simulink library "amg_high_precision_rtc"  (R2015b)
settings: Solver=ode45  StartTime=0.0  StopTime=10.0  RelTol=1e-3
libraries: simulink x207, waijung_soft_i2c_lib x11, amg_high_precision_rtc x10
(part 3 of 5)

== system amg_high_precision_rtc/STM32F4/DS3231 Get Time/Convert/Convert Hour ==
  In1 : Inport
  Add : Sum
  Constant : Constant  Value=10  OutDataTypeStr=uint8
  Extract Bits : simulink/Logic and Bit Operations/Extract Bits  SystemSampleTime=-1  bitsToExtract=Range of bits  numBits=8  bitIdxRange=[4 5]  outScalingMode=Treat bit field as an integer
  Extract Bits1 : simulink/Logic and Bit Operations/Extract Bits  SystemSampleTime=-1  bitsToExtract=Range of bits  numBits=8  bitIdxRange=[0 3]  outScalingMode=Treat bit field as an integer
  Extract Bits2 : simulink/Logic and Bit Operations/Extract Bits  SystemSampleTime=-1  bitsToExtract=Range of bits  numBits=8  bitIdxRange=[5 5]  outScalingMode=Treat bit field as an integer
  Product : Product  RndMeth=Zero
  Hour : Outport
  AM/PM : Outport  Port=2
  wires:
  Add/1 -> Hour/1
  Product/1 -> Add/1
  Extract Bits/1 -> Product/2
  Constant/1 -> Product/1
  In1/1 -> Extract Bits/1, Extract Bits1/1, Extract Bits2/1
  Extract Bits1/1 -> Add/2
  Extract Bits2/1 -> AM/PM/1

== system amg_high_precision_rtc/STM32F4/DS3231 Get Time/Convert/Convert Second// Minute ==
  In1 : Inport
  Add : Sum
  Constant : Constant  Value=10  OutDataTypeStr=uint8
  Extract Bits : simulink/Logic and Bit Operations/Extract Bits  SystemSampleTime=-1  bitsToExtract=Range of bits  numBits=8  bitIdxRange=[4 6]  outScalingMode=Treat bit field as an integer
  Extract Bits1 : simulink/Logic and Bit Operations/Extract Bits  SystemSampleTime=-1  bitsToExtract=Range of bits  numBits=8  bitIdxRange=[0 3]  outScalingMode=Treat bit field as an integer
  Product : Product  RndMeth=Zero
  Out1 : Outport
  wires:
  In1/1 -> Extract Bits/1, Extract Bits1/1
  Constant/1 -> Product/1
  Extract Bits/1 -> Product/2
  Product/1 -> Add/1
  Extract Bits1/1 -> Add/2
  Add/1 -> Out1/1

== system amg_high_precision_rtc/STM32F4/DS3231Temperture/Check Busy// Write Conv/If Action Active CONV ==
  In1 : Inport
  Action Port : ActionPort  PropagateVarSize=During execution  ActionType=then
  CONV : Constant  Value=hex2dec('3C')  OutDataTypeStr=uint8
  I2C Master Read/Write1 : S-Function  FunctionName=stm32f4_i2c  Parameters=configuration,module,transfer,clkspeed,timeout,sdapin,sclpin,writecount,readcount,inputtypearray,outputtypearray,confstr,sampletime,sampletimestr,blockid  SFunctionDeploymentMode=off  EnableBusSupport=off  mask(stm32f4_i2c){configuration=Transaction, module=1, lastmodule=3, transfer=Blocking, dutycycle=TLow/THigh = 2, clkspeed=400, timeout=25, writecount=2, readcount=0, sdapin=C9, sclpin=A8, waitwritetime=0, inputtypearray=[3 3 3 3], outputtypearray=[1 3], confstr=["C","9","A","8","1","1","6","0","I2C_DutyCycle_2","0"], sampletime=-1, sampletimestr=0, blockid=amg_high_precision_rtcTempertureReadSubsystemIfActionSubsystemI2CMasterReadWrite1}
      mask prompts: module "I2C Module"; lastmodule "Last module"; transfer "Transfer mode"; dutycycle "Duty cycle in fast mode"; clkspeed "Clock speed (kHz)"; timeout "Timeout (ms)"; writecount "Bytes write count"; readcount "Bytes read count"; sdapin "SDA pin"; sclpin "SCL pin"; waitwritetime "Wait write time (ms), default is 0"; inputtypearray "Input type array"; outputtypearray "Output type array"; confstr "Configuration string"; sampletime "Sample time (sec)"; sampletimestr "Compiled sample time (sec) in string"
      mask init:
      | stm32f4_i2c_callback('init');
      mask Help: web(fullfile(waijungdocroot,'stm32f4_i2c_readwrite.htm'), '-browser')
      mask TypeOptions configuration: Setup | Transaction
      mask Callback configuration: stm32f4_i2c_callback('configuration');
      mask TypeOptions module: 1 | 2 | 3
      mask Callback module: stm32f4_i2c_callback('module');
      mask TypeOptions transfer: Blocking | Non-blocking
      mask TypeOptions dutycycle: TLow/THigh = 16/9 | TLow/THigh = 2
      mask Callback dutycycle: stm32f4_i2c_callback('dutycycle');
      mask Callback writecount: stm32f4_i2c_callback('writecount');
      mask Callback readcount: stm32f4_i2c_callback('readcount');
      mask TypeOptions sdapin: - | C9
      mask Callback sdapin: stm32f4_i2c_callback('sdapin');
      mask TypeOptions sclpin: - | A8
      mask Callback sclpin: stm32f4_i2c_callback('sclpin');
      mask Callback confstr: stm32f4_i2c_callback('confstr');
      mask Callback sampletime: stm32f4_i2c_callback('sampletime');
      mask Callback sampletimestr: stm32f4_i2c_callback('sampletimestr');
      mask Callback blockid: stm32f4_i2c_callback('blockid');
      mask Display: text(0.5, 0.5, 'Module: I2C1\nTransfer: Blocking\nWrite: 2 bytes\nRead: 0 bytes\nTs (sec): 0','ver','middle','hor','center');port_label('input', 1,'SlvAddr');port_label('input', 2,'Wr0 (uint8)');port_label('input', 3,'Wr1 (uint8)');port_label('output', 1,'Status');
  REG_CNTRL : Constant  Value=hex2dec('0E')  OutDataTypeStr=uint8
  Terminator : Terminator
  wires:
  In1/1 -> I2C Master Read/Write1/1
  CONV/1 -> I2C Master Read/Write1/3
  REG_CNTRL/1 -> I2C Master Read/Write1/2
  I2C Master Read/Write1/1 -> Terminator/1

== system amg_high_precision_rtc/Soft I2C/Soft-DS3231 Configure/Debouce4/Enabled Subsystem ==
  Enable : EnablePort  PropagateVarSize=During execution
  Counter Free-Running : simulink/Sources/Counter Free-Running  SystemSampleTime=-1  NumBits=32  tsamp=-1
  Out1 : Outport  InitialOutput=0
  wires:
  Counter Free-Running/1 -> Out1/1

== system amg_high_precision_rtc/Soft I2C/Soft-DS3231 Configure/Debouce4/Enabled Subsystem1 ==
  Enable : EnablePort  PropagateVarSize=During execution
  Bitwise Operator : simulink/Logic and Bit Operations/Bitwise Operator  logicop=AND  UseBitMask=on  BitMask=1  BitMaskRealWorld=Stored Integer
  Compare To Zero : simulink/Logic and Bit Operations/Compare To Zero  SystemSampleTime=-1  relop===  LogicOutDataTypeMode=uint8  ZeroCross=off
  Counter Free-Running : simulink/Sources/Counter Free-Running  SystemSampleTime=-1  NumBits=32  tsamp=-1
  Out1 : Outport  InitialOutput=0
  wires:
  Compare To Zero/1 -> Out1/1
  Bitwise Operator/1 -> Compare To Zero/1
  Counter Free-Running/1 -> Bitwise Operator/1

== system amg_high_precision_rtc/Soft I2C/Soft-DS3231 Configure/Debouce4/Enabled Subsystem4 ==
  Enable : EnablePort  PropagateVarSize=During execution
  Counter Free-Running : simulink/Sources/Counter Free-Running  SystemSampleTime=-1  NumBits=32  tsamp=-1
  Out1 : Outport  InitialOutput=0
  wires:
  Counter Free-Running/1 -> Out1/1

== system amg_high_precision_rtc/Soft I2C/Soft-DS3231 Configure/Debouce4/Enabled Subsystem5 ==
  Enable : EnablePort  PropagateVarSize=During execution
  Counter Free-Running : simulink/Sources/Counter Free-Running  SystemSampleTime=-1  NumBits=32  tsamp=-1
  Out1 : Outport  InitialOutput=0
  wires:
  Counter Free-Running/1 -> Out1/1

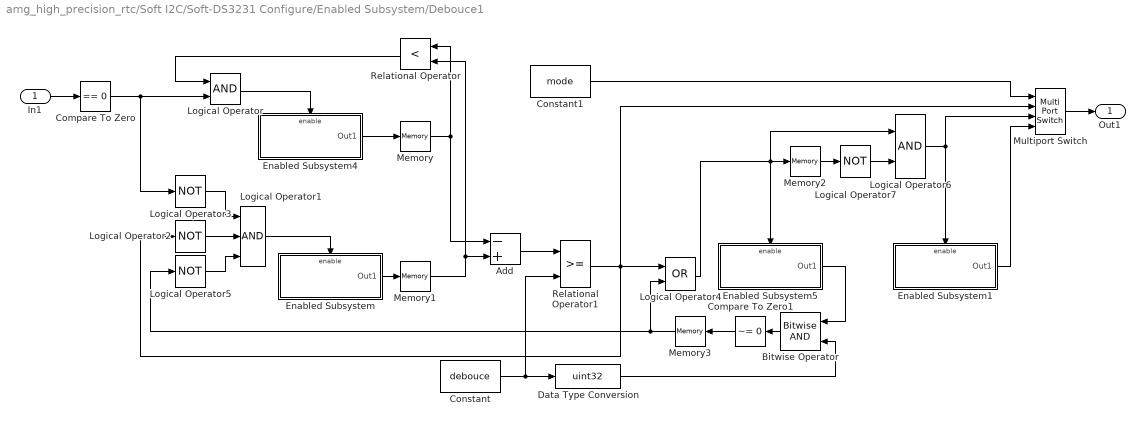
== system amg_high_precision_rtc/Soft I2C/Soft-DS3231 Configure/Enabled Subsystem/Debouce1 ==
  In1 : Inport
  Add : Sum  Inputs=-+  OutDataTypeStr=int32
  Bitwise Operator : simulink/Logic and Bit Operations/Bitwise Operator  logicop=AND  UseBitMask=off  NumInputPorts=2  BitMask=debouce  BitMaskRealWorld=Stored Integer
  Compare To Zero : simulink/Logic and Bit Operations/Compare To Zero  SystemSampleTime=-1  relop===  LogicOutDataTypeMode=uint8  ZeroCross=off
  Compare To Zero1 : simulink/Logic and Bit Operations/Compare To Zero  SystemSampleTime=-1  relop=~=  LogicOutDataTypeMode=boolean  ZeroCross=off
  Constant : Constant  Value=debouce  OutDataTypeStr=int32
  Constant1 : Constant  Value=mode  OutDataTypeStr=int32
  Data Type Conversion : DataTypeConversion  OutDataTypeStr=uint32
  Enabled Subsystem : Subsystem  TreatAsAtomicUnit=on
  Enabled Subsystem1 : Subsystem  TreatAsAtomicUnit=on
  Enabled Subsystem4 : Subsystem  TreatAsAtomicUnit=on
  Enabled Subsystem5 : Subsystem  TreatAsAtomicUnit=on
  Logical Operator : Logic  AllPortsSameDT=off  OutDataTypeStr=boolean
  Logical Operator1 : Logic  Inputs=3  AllPortsSameDT=off  OutDataTypeStr=boolean
  Logical Operator{2..3,5,7} (4 alike) : Logic  Operator=NOT  AllPortsSameDT=off  OutDataTypeStr=boolean
  Logical Operator4 : Logic  Operator=OR  AllPortsSameDT=off  OutDataTypeStr=boolean
  Logical Operator6 : Logic  AllPortsSameDT=off  OutDataTypeStr=boolean
  Memory{,1..3} (4 alike) : Memory  LinearizeMemory=on
  Multiport Switch : MultiPortSwitch
  Relational Operator : RelationalOperator  Operator=<  OutDataTypeStr=boolean
  Relational Operator1 : RelationalOperator  OutDataTypeStr=boolean  InputSameDT=on
  Out1 : Outport
  wires:
  Logical Operator1/1 -> Enabled Subsystem/Enable
  Relational Operator1/1 -> Logical Operator2/1, Logical Operator4/1, Multiport Switch/2
  Logical Operator7/1 -> Logical Operator6/2
  Memory2/1 -> Logical Operator7/1
  Logical Operator4/1 -> Logical Operator6/1, Memory2/1, Enabled Subsystem5/Enable
  Enabled Subsystem5/1(Out1) -> Bitwise Operator/1
  Bitwise Operator/1 -> Compare To Zero1/1
  Compare To Zero1/1 -> Memory3/1
  Logical Operator3/1 -> Logical Operator1/1
  Logical Operator5/1 -> Logical Operator1/3
  Memory3/1 -> Logical Operator5/1, Logical Operator4/2
  Logical Operator2/1 -> Logical Operator1/2
  Constant/1 -> Relational Operator1/2, Data Type Conversion/1
  Add/1 -> Relational Operator1/1
  Relational Operator/1 -> Logical Operator/1
  Logical Operator/1 -> Enabled Subsystem4/Enable
  Compare To Zero/1 -> Logical Operator3/1, Logical Operator/2
  Memory1/1 -> Relational Operator/2, Add/2
  Memory/1 -> Add/1, Relational Operator/1
  Enabled Subsystem4/1(Out1) -> Memory/1
  Enabled Subsystem/1(Out1) -> Memory1/1
  In1/1 -> Compare To Zero/1
  Logical Operator6/1 -> Multiport Switch/3, Enabled Subsystem1/Enable
  Enabled Subsystem1/1(Out1) -> Multiport Switch/4
  Data Type Conversion/1 -> Bitwise Operator/2
  Multiport Switch/1 -> Out1/1
  Constant1/1 -> Multiport Switch/1

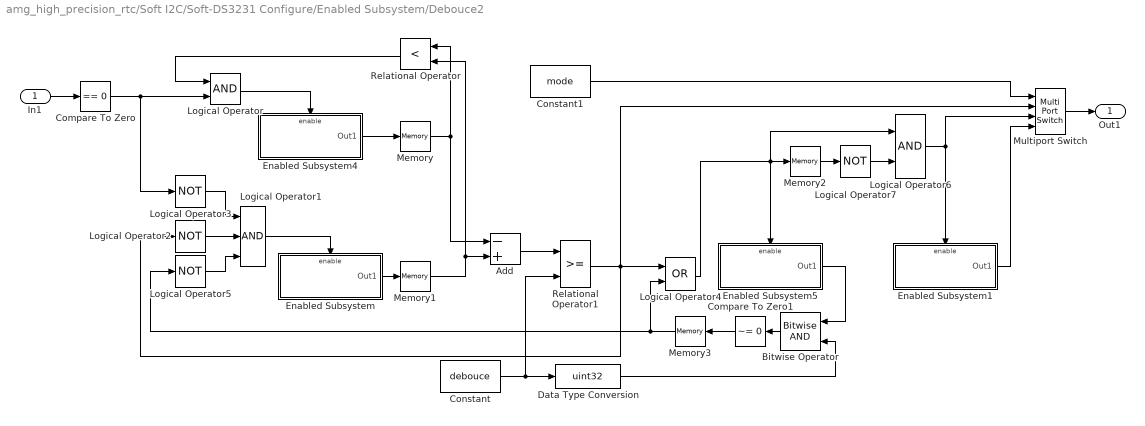
== system amg_high_precision_rtc/Soft I2C/Soft-DS3231 Configure/Enabled Subsystem/Debouce2 ==
  In1 : Inport
  Add : Sum  Inputs=-+  OutDataTypeStr=int32
  Bitwise Operator : simulink/Logic and Bit Operations/Bitwise Operator  logicop=AND  UseBitMask=off  NumInputPorts=2  BitMask=debouce  BitMaskRealWorld=Stored Integer
  Compare To Zero : simulink/Logic and Bit Operations/Compare To Zero  SystemSampleTime=-1  relop===  LogicOutDataTypeMode=uint8  ZeroCross=off
  Compare To Zero1 : simulink/Logic and Bit Operations/Compare To Zero  SystemSampleTime=-1  relop=~=  LogicOutDataTypeMode=boolean  ZeroCross=off
  Constant : Constant  Value=debouce  OutDataTypeStr=int32
  Constant1 : Constant  Value=mode  OutDataTypeStr=int32
  Data Type Conversion : DataTypeConversion  OutDataTypeStr=uint32
  Enabled Subsystem : Subsystem  TreatAsAtomicUnit=on
  Enabled Subsystem1 : Subsystem  TreatAsAtomicUnit=on
  Enabled Subsystem4 : Subsystem  TreatAsAtomicUnit=on
  Enabled Subsystem5 : Subsystem  TreatAsAtomicUnit=on
  Logical Operator : Logic  AllPortsSameDT=off  OutDataTypeStr=boolean
  Logical Operator1 : Logic  Inputs=3  AllPortsSameDT=off  OutDataTypeStr=boolean
  Logical Operator{2..3,5,7} (4 alike) : Logic  Operator=NOT  AllPortsSameDT=off  OutDataTypeStr=boolean
  Logical Operator4 : Logic  Operator=OR  AllPortsSameDT=off  OutDataTypeStr=boolean
  Logical Operator6 : Logic  AllPortsSameDT=off  OutDataTypeStr=boolean
  Memory{,1..3} (4 alike) : Memory  LinearizeMemory=on
  Multiport Switch : MultiPortSwitch
  Relational Operator : RelationalOperator  Operator=<  OutDataTypeStr=boolean
  Relational Operator1 : RelationalOperator  OutDataTypeStr=boolean  InputSameDT=on
  Out1 : Outport
  wires:
  Logical Operator1/1 -> Enabled Subsystem/Enable
  Relational Operator1/1 -> Logical Operator2/1, Logical Operator4/1, Multiport Switch/2
  Logical Operator7/1 -> Logical Operator6/2
  Memory2/1 -> Logical Operator7/1
  Logical Operator4/1 -> Logical Operator6/1, Memory2/1, Enabled Subsystem5/Enable
  Enabled Subsystem5/1(Out1) -> Bitwise Operator/1
  Bitwise Operator/1 -> Compare To Zero1/1
  Compare To Zero1/1 -> Memory3/1
  Logical Operator3/1 -> Logical Operator1/1
  Logical Operator5/1 -> Logical Operator1/3
  Memory3/1 -> Logical Operator5/1, Logical Operator4/2
  Logical Operator2/1 -> Logical Operator1/2
  Constant/1 -> Relational Operator1/2, Data Type Conversion/1
  Add/1 -> Relational Operator1/1
  Relational Operator/1 -> Logical Operator/1
  Logical Operator/1 -> Enabled Subsystem4/Enable
  Compare To Zero/1 -> Logical Operator3/1, Logical Operator/2
  Memory1/1 -> Relational Operator/2, Add/2
  Memory/1 -> Add/1, Relational Operator/1
  Enabled Subsystem4/1(Out1) -> Memory/1
  Enabled Subsystem/1(Out1) -> Memory1/1
  In1/1 -> Compare To Zero/1
  Logical Operator6/1 -> Multiport Switch/3, Enabled Subsystem1/Enable
  Enabled Subsystem1/1(Out1) -> Multiport Switch/4
  Data Type Conversion/1 -> Bitwise Operator/2
  Multiport Switch/1 -> Out1/1
  Constant1/1 -> Multiport Switch/1

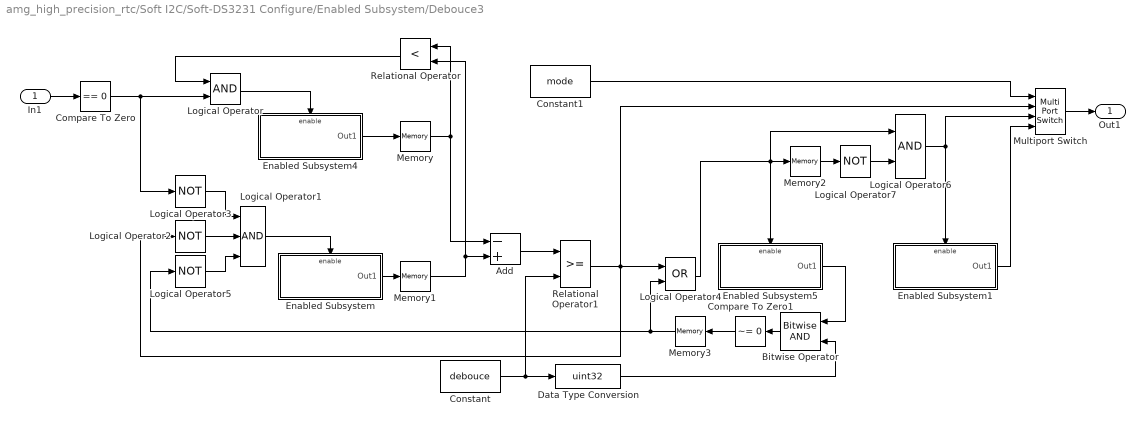
== system amg_high_precision_rtc/Soft I2C/Soft-DS3231 Configure/Enabled Subsystem/Debouce3 ==
  In1 : Inport
  Add : Sum  Inputs=-+  OutDataTypeStr=int32
  Bitwise Operator : simulink/Logic and Bit Operations/Bitwise Operator  logicop=AND  UseBitMask=off  NumInputPorts=2  BitMask=debouce  BitMaskRealWorld=Stored Integer
  Compare To Zero : simulink/Logic and Bit Operations/Compare To Zero  SystemSampleTime=-1  relop===  LogicOutDataTypeMode=uint8  ZeroCross=off
  Compare To Zero1 : simulink/Logic and Bit Operations/Compare To Zero  SystemSampleTime=-1  relop=~=  LogicOutDataTypeMode=boolean  ZeroCross=off
  Constant : Constant  Value=debouce  OutDataTypeStr=int32
  Constant1 : Constant  Value=mode  OutDataTypeStr=int32
  Data Type Conversion : DataTypeConversion  OutDataTypeStr=uint32
  Enabled Subsystem : Subsystem  TreatAsAtomicUnit=on
  Enabled Subsystem1 : Subsystem  TreatAsAtomicUnit=on
  Enabled Subsystem4 : Subsystem  TreatAsAtomicUnit=on
  Enabled Subsystem5 : Subsystem  TreatAsAtomicUnit=on
  Logical Operator : Logic  AllPortsSameDT=off  OutDataTypeStr=boolean
  Logical Operator1 : Logic  Inputs=3  AllPortsSameDT=off  OutDataTypeStr=boolean
  Logical Operator{2..3,5,7} (4 alike) : Logic  Operator=NOT  AllPortsSameDT=off  OutDataTypeStr=boolean
  Logical Operator4 : Logic  Operator=OR  AllPortsSameDT=off  OutDataTypeStr=boolean
  Logical Operator6 : Logic  AllPortsSameDT=off  OutDataTypeStr=boolean
  Memory{,1..3} (4 alike) : Memory  LinearizeMemory=on
  Multiport Switch : MultiPortSwitch
  Relational Operator : RelationalOperator  Operator=<  OutDataTypeStr=boolean
  Relational Operator1 : RelationalOperator  OutDataTypeStr=boolean  InputSameDT=on
  Out1 : Outport
  wires:
  Logical Operator1/1 -> Enabled Subsystem/Enable
  Relational Operator1/1 -> Logical Operator2/1, Logical Operator4/1, Multiport Switch/2
  Logical Operator7/1 -> Logical Operator6/2
  Memory2/1 -> Logical Operator7/1
  Logical Operator4/1 -> Logical Operator6/1, Memory2/1, Enabled Subsystem5/Enable
  Enabled Subsystem5/1(Out1) -> Bitwise Operator/1
  Bitwise Operator/1 -> Compare To Zero1/1
  Compare To Zero1/1 -> Memory3/1
  Logical Operator3/1 -> Logical Operator1/1
  Logical Operator5/1 -> Logical Operator1/3
  Memory3/1 -> Logical Operator5/1, Logical Operator4/2
  Logical Operator2/1 -> Logical Operator1/2
  Constant/1 -> Relational Operator1/2, Data Type Conversion/1
  Add/1 -> Relational Operator1/1
  Relational Operator/1 -> Logical Operator/1
  Logical Operator/1 -> Enabled Subsystem4/Enable
  Compare To Zero/1 -> Logical Operator3/1, Logical Operator/2
  Memory1/1 -> Relational Operator/2, Add/2
  Memory/1 -> Add/1, Relational Operator/1
  Enabled Subsystem4/1(Out1) -> Memory/1
  Enabled Subsystem/1(Out1) -> Memory1/1
  In1/1 -> Compare To Zero/1
  Logical Operator6/1 -> Multiport Switch/3, Enabled Subsystem1/Enable
  Enabled Subsystem1/1(Out1) -> Multiport Switch/4
  Data Type Conversion/1 -> Bitwise Operator/2
  Multiport Switch/1 -> Out1/1
  Constant1/1 -> Multiport Switch/1

== system amg_high_precision_rtc/Soft I2C/Soft-DS3231 Configure/Enabled Subsystem/Generate Mode ID ==
  note: # check unused state
  In1 : Inport
  Compare To Constant : simulink/Logic and Bit Operations/Compare To Constant  SystemSampleTime=-1  relop=>  const=5  LogicOutDataTypeMode=boolean  ZeroCross=off
  Enabled Subsystem2 : Subsystem  TreatAsAtomicUnit=on
  Logical Operator : Logic  Operator=OR  AllPortsSameDT=off  OutDataTypeStr=boolean
  Unit Delay : UnitDelay  SampleTime=-1
  Out1 : Outport
  wires:
  In1/1 -> Logical Operator/2
  Unit Delay/1 -> Compare To Constant/1
  Compare To Constant/1 -> Logical Operator/1
  Logical Operator/1 -> Enabled Subsystem2/Enable
  Enabled Subsystem2/1(Out1) -> Out1/1, Unit Delay/1

== system amg_high_precision_rtc/Soft I2C/Soft-DS3231 Configure/Enabled Subsystem/Subsystem ==
  Up : Inport
  Down : Inport  Port=2
  SlvAddr : Inport  Port=3
  Adjust State : Inport  Port=4
  Enable : EnablePort  PropagateVarSize=During execution
  Enabled Subsystem : Subsystem  TreatAsAtomicUnit=on
  Logical Operator : Logic  AllPortsSameDT=off  OutDataTypeStr=boolean
  Soft-DS3231 Get Date : Subsystem  mask(amg_high_precision_rtc){blockfunction=date, module=1}
      mask prompts: blockfunction "Function"; module "I2C module"
      mask init:
      | amg_high_precision_rtc_callback('init');
      mask Help: web(fullfile(waijungdocroot,'DS3231_Get_Date.htm'), '-browser')
      mask TypeOptions blockfunction: temp | time | date
      mask TypeOptions module: 1 | 2 | 3 | 4 | 5 | 6 | 7 | 8 | 9 | 10 | 11 | 12 | 13 | 14 | 15 | 16 | 17 | 18 | 19 | 20 | 21 | 22 | 23 | 24 | 25 | 26 | 27 | 28 | 29 | 30 | 31 | 32
      mask Callback module: amg_high_precision_rtc_callback('module');
      mask Display: text(0.5, 0.5, 'Port: I2C1','ver','middle','hor','center');port_label('input', 1,'SlvAddr');port_label('output', 1,'Status');port_label('output', 2,'Day(1-7)');port_label('output', 3,'Date(1-31)');port_label('output', 4,'Month(1-12)');port_label('output', 5,'Year(0-99)');
  Soft-DS3231 Get Time : Subsystem  mask(amg_high_precision_rtc){blockfunction=time, module=1}
      mask prompts: blockfunction "Function"; module "I2C module"
      mask init:
      | amg_high_precision_rtc_callback('init');
      mask Help: web(fullfile(waijungdocroot,'DS3231_Get_Time.htm'), '-browser')
      mask TypeOptions blockfunction: temp | time | date
      mask TypeOptions module: 1 | 2 | 3 | 4 | 5 | 6 | 7 | 8 | 9 | 10 | 11 | 12 | 13 | 14 | 15 | 16 | 17 | 18 | 19 | 20 | 21 | 22 | 23 | 24 | 25 | 26 | 27 | 28 | 29 | 30 | 31 | 32
      mask Callback module: amg_high_precision_rtc_callback('module');
      mask Display: text(0.5, 0.5, 'Port: I2C1','ver','middle','hor','center');port_label('input', 1,'SlvAddr');port_label('output', 1,'Status');port_label('output', 2,'Hour(0-11/23)');port_label('output', 3,'Minute(0-59)');port_label('output', 4,'Second(0-59)');port_label('output', 5,'AM(0)/PM(1)');
  Terminator : Terminator
  Terminator1 : Terminator
  wires:
  Soft-DS3231 Get Time/1(Status) -> Logical Operator/2
  Soft-DS3231 Get Date/1(Status) -> Logical Operator/1
  Logical Operator/1 -> Enabled Subsystem/Enable
  Soft-DS3231 Get Time/5(AM/PM) -> Terminator1/1
  Soft-DS3231 Get Date/3(Date) -> Enabled Subsystem/1(dd)
  Soft-DS3231 Get Time/4(Second) -> Enabled Subsystem/6(ss)
  Soft-DS3231 Get Time/3(Minute) -> Enabled Subsystem/5(mi)
  Soft-DS3231 Get Time/2(Hour) -> Enabled Subsystem/4(hh)
  Down/1 -> Enabled Subsystem/9(down)
  Up/1 -> Enabled Subsystem/8(up)
  Adjust State/1 -> Enabled Subsystem/7(adjust state)
  Soft-DS3231 Get Date/2(Day) -> Terminator/1
  SlvAddr/1 -> Enabled Subsystem/10(SlvAddr), Soft-DS3231 Get Time/1(Slave Address), Soft-DS3231 Get Date/1(Slave Address)
  Soft-DS3231 Get Date/5(Year) -> Enabled Subsystem/3(yy)
  Soft-DS3231 Get Date/4(Month) -> Enabled Subsystem/2(mm)

== system amg_high_precision_rtc/Soft I2C/Soft-DS3231 Get Date/Convert/Convert 1 ==
  In1 : Inport
  Add : Sum
  Constant : Constant  Value=10  OutDataTypeStr=uint8
  Extract Bits : simulink/Logic and Bit Operations/Extract Bits  SystemSampleTime=-1  bitsToExtract=Range of bits  numBits=8  bitIdxRange=[4 5]  outScalingMode=Treat bit field as an integer
  Extract Bits1 : simulink/Logic and Bit Operations/Extract Bits  SystemSampleTime=-1  bitsToExtract=Range of bits  numBits=8  bitIdxRange=[0 3]  outScalingMode=Treat bit field as an integer
  Product : Product  RndMeth=Zero
  Out1 : Outport
  wires:
  Add/1 -> Out1/1
  Extract Bits1/1 -> Add/2
  Product/1 -> Add/1
  Extract Bits/1 -> Product/2
  Constant/1 -> Product/1
  In1/1 -> Extract Bits1/1, Extract Bits/1

== system amg_high_precision_rtc/Soft I2C/Soft-DS3231 Get Date/Convert/Convert 2 ==
  In1 : Inport
  Add : Sum
  Constant : Constant  Value=10  OutDataTypeStr=uint8
  Extract Bits : simulink/Logic and Bit Operations/Extract Bits  SystemSampleTime=-1  bitsToExtract=Range of bits  numBits=8  bitIdxRange=[4 4]  outScalingMode=Treat bit field as an integer
  Extract Bits1 : simulink/Logic and Bit Operations/Extract Bits  SystemSampleTime=-1  bitsToExtract=Range of bits  numBits=8  bitIdxRange=[0 3]  outScalingMode=Treat bit field as an integer
  Product : Product  RndMeth=Zero
  Out1 : Outport
  wires:
  In1/1 -> Extract Bits/1, Extract Bits1/1
  Constant/1 -> Product/1
  Extract Bits/1 -> Product/2
  Product/1 -> Add/1
  Extract Bits1/1 -> Add/2
  Add/1 -> Out1/1

== system amg_high_precision_rtc/Soft I2C/Soft-DS3231 Get Date/Convert/Convert 3 ==
  In1 : Inport
  Add : Sum
  Constant : Constant  Value=10  OutDataTypeStr=uint8
  Extract Bits : simulink/Logic and Bit Operations/Extract Bits  SystemSampleTime=-1  bitsToExtract=Range of bits  numBits=8  bitIdxRange=[4 7]  outScalingMode=Treat bit field as an integer
  Extract Bits1 : simulink/Logic and Bit Operations/Extract Bits  SystemSampleTime=-1  bitsToExtract=Range of bits  numBits=8  bitIdxRange=[0 3]  outScalingMode=Treat bit field as an integer
  Product : Product  RndMeth=Zero
  Out1 : Outport
  wires:
  Add/1 -> Out1/1
  Extract Bits1/1 -> Add/2
  Product/1 -> Add/1
  Extract Bits/1 -> Product/2
  Constant/1 -> Product/1
  In1/1 -> Extract Bits1/1, Extract Bits/1

== system amg_high_precision_rtc/Soft I2C/Soft-DS3231 Get Time/Convert/Convert Hour ==
  In1 : Inport
  Add : Sum
  Constant : Constant  Value=10  OutDataTypeStr=uint8
  Extract Bits : simulink/Logic and Bit Operations/Extract Bits  SystemSampleTime=-1  bitsToExtract=Range of bits  numBits=8  bitIdxRange=[4 5]  outScalingMode=Treat bit field as an integer
  Extract Bits1 : simulink/Logic and Bit Operations/Extract Bits  SystemSampleTime=-1  bitsToExtract=Range of bits  numBits=8  bitIdxRange=[0 3]  outScalingMode=Treat bit field as an integer
  Extract Bits2 : simulink/Logic and Bit Operations/Extract Bits  SystemSampleTime=-1  bitsToExtract=Range of bits  numBits=8  bitIdxRange=[5 5]  outScalingMode=Treat bit field as an integer
  Product : Product  RndMeth=Zero
  Hour : Outport
  AM/PM : Outport  Port=2
  wires:
  Extract Bits2/1 -> AM/PM/1
  Extract Bits1/1 -> Add/2
  In1/1 -> Extract Bits2/1, Extract Bits1/1, Extract Bits/1
  Constant/1 -> Product/1
  Extract Bits/1 -> Product/2
  Product/1 -> Add/1
  Add/1 -> Hour/1

== system amg_high_precision_rtc/Soft I2C/Soft-DS3231 Get Time/Convert/Convert Second// Minute ==
  In1 : Inport
  Add : Sum
  Constant : Constant  Value=10  OutDataTypeStr=uint8
  Extract Bits : simulink/Logic and Bit Operations/Extract Bits  SystemSampleTime=-1  bitsToExtract=Range of bits  numBits=8  bitIdxRange=[4 6]  outScalingMode=Treat bit field as an integer
  Extract Bits1 : simulink/Logic and Bit Operations/Extract Bits  SystemSampleTime=-1  bitsToExtract=Range of bits  numBits=8  bitIdxRange=[0 3]  outScalingMode=Treat bit field as an integer
  Product : Product  RndMeth=Zero
  Out1 : Outport
  wires:
  Add/1 -> Out1/1
  Extract Bits1/1 -> Add/2
  Product/1 -> Add/1
  Extract Bits/1 -> Product/2
  Constant/1 -> Product/1
  In1/1 -> Extract Bits1/1, Extract Bits/1

== system amg_high_precision_rtc/Soft I2C/Soft-DS3231Temperture/Check Busy// Write Conv/If Action Active CONV ==
  In1 : Inport
  Action Port : ActionPort  PropagateVarSize=During execution  ActionType=then
  CONV : Constant  Value=hex2dec('3C')  OutDataTypeStr=uint8
  REG_CNTRL : Constant  Value=hex2dec('0E')  OutDataTypeStr=uint8
  Soft I2C Master Read/Write : waijung_soft_i2c_lib/Soft I2C Master Read//Write  conf=ReadWrite  targetname=0  module=1  transfer=Blocking  clk=100  timeout=25  sdapins={'A4','A6'}  sclpins='A5'  writecount=2  readcount=0  waittime=0  forcestop=off  portpinstr=0  sampletime=-1  blockid=SoftI2CSoftDS3231TempertureCheckBusyWriteConvIfActionActiveCONVSoftI2CMasterReadWrite  inputporttype=[3 3 3]  inputportwidth=[]  inputportlabel={'SlvAddr' 'Wr0 (uint8)' 'Wr1 (uint8)'}  outputporttype=[3]  outputportwidth=[1]  outputportlabel={'Status'}  compat=0  optionstring=[]
  Terminator : Terminator
  wires:
  Soft I2C Master Read/Write/1 -> Terminator/1
  REG_CNTRL/1 -> Soft I2C Master Read/Write/2
  CONV/1 -> Soft I2C Master Read/Write/3
  In1/1 -> Soft I2C Master Read/Write/1

== system amg_high_precision_rtc/STM32F4/DS3231 Configure/Enabled Subsystem/Debouce1/Enabled Subsystem ==
  Enable : EnablePort  PropagateVarSize=During execution
  Counter Free-Running : simulink/Sources/Counter Free-Running  SystemSampleTime=-1  NumBits=32  tsamp=-1
  Out1 : Outport  InitialOutput=0
  wires:
  Counter Free-Running/1 -> Out1/1

== system amg_high_precision_rtc/STM32F4/DS3231 Configure/Enabled Subsystem/Debouce1/Enabled Subsystem1 ==
  Enable : EnablePort  PropagateVarSize=During execution
  Bitwise Operator : simulink/Logic and Bit Operations/Bitwise Operator  logicop=AND  UseBitMask=on  BitMask=1  BitMaskRealWorld=Stored Integer
  Compare To Zero : simulink/Logic and Bit Operations/Compare To Zero  SystemSampleTime=-1  relop===  LogicOutDataTypeMode=uint8  ZeroCross=off
  Counter Free-Running : simulink/Sources/Counter Free-Running  SystemSampleTime=-1  NumBits=32  tsamp=-1
  Out1 : Outport  InitialOutput=0
  wires:
  Counter Free-Running/1 -> Bitwise Operator/1
  Bitwise Operator/1 -> Compare To Zero/1
  Compare To Zero/1 -> Out1/1

== system amg_high_precision_rtc/STM32F4/DS3231 Configure/Enabled Subsystem/Debouce1/Enabled Subsystem4 ==
  Enable : EnablePort  PropagateVarSize=During execution
  Counter Free-Running : simulink/Sources/Counter Free-Running  SystemSampleTime=-1  NumBits=32  tsamp=-1
  Out1 : Outport  InitialOutput=0
  wires:
  Counter Free-Running/1 -> Out1/1

== system amg_high_precision_rtc/STM32F4/DS3231 Configure/Enabled Subsystem/Debouce1/Enabled Subsystem5 ==
  Enable : EnablePort  PropagateVarSize=During execution
  Counter Free-Running : simulink/Sources/Counter Free-Running  SystemSampleTime=-1  NumBits=32  tsamp=-1
  Out1 : Outport  InitialOutput=0
  wires:
  Counter Free-Running/1 -> Out1/1

== system amg_high_precision_rtc/STM32F4/DS3231 Configure/Enabled Subsystem/Debouce2/Enabled Subsystem ==
  Enable : EnablePort  PropagateVarSize=During execution
  Counter Free-Running : simulink/Sources/Counter Free-Running  SystemSampleTime=-1  NumBits=32  tsamp=-1
  Out1 : Outport  InitialOutput=0
  wires:
  Counter Free-Running/1 -> Out1/1

== system amg_high_precision_rtc/STM32F4/DS3231 Configure/Enabled Subsystem/Debouce2/Enabled Subsystem1 ==
  Enable : EnablePort  PropagateVarSize=During execution
  Bitwise Operator : simulink/Logic and Bit Operations/Bitwise Operator  logicop=AND  UseBitMask=on  BitMask=1  BitMaskRealWorld=Stored Integer
  Compare To Zero : simulink/Logic and Bit Operations/Compare To Zero  SystemSampleTime=-1  relop===  LogicOutDataTypeMode=uint8  ZeroCross=off
  Counter Free-Running : simulink/Sources/Counter Free-Running  SystemSampleTime=-1  NumBits=32  tsamp=-1
  Out1 : Outport  InitialOutput=0
  wires:
  Counter Free-Running/1 -> Bitwise Operator/1
  Bitwise Operator/1 -> Compare To Zero/1
  Compare To Zero/1 -> Out1/1

== system amg_high_precision_rtc/STM32F4/DS3231 Configure/Enabled Subsystem/Debouce2/Enabled Subsystem4 ==
  Enable : EnablePort  PropagateVarSize=During execution
  Counter Free-Running : simulink/Sources/Counter Free-Running  SystemSampleTime=-1  NumBits=32  tsamp=-1
  Out1 : Outport  InitialOutput=0
  wires:
  Counter Free-Running/1 -> Out1/1

== system amg_high_precision_rtc/STM32F4/DS3231 Configure/Enabled Subsystem/Debouce2/Enabled Subsystem5 ==
  Enable : EnablePort  PropagateVarSize=During execution
  Counter Free-Running : simulink/Sources/Counter Free-Running  SystemSampleTime=-1  NumBits=32  tsamp=-1
  Out1 : Outport  InitialOutput=0
  wires:
  Counter Free-Running/1 -> Out1/1

== system amg_high_precision_rtc/STM32F4/DS3231 Configure/Enabled Subsystem/Debouce3/Enabled Subsystem ==
  Enable : EnablePort  PropagateVarSize=During execution
  Counter Free-Running : simulink/Sources/Counter Free-Running  SystemSampleTime=-1  NumBits=32  tsamp=-1
  Out1 : Outport  InitialOutput=0
  wires:
  Counter Free-Running/1 -> Out1/1

== system amg_high_precision_rtc/STM32F4/DS3231 Configure/Enabled Subsystem/Debouce3/Enabled Subsystem1 ==
  Enable : EnablePort  PropagateVarSize=During execution
  Bitwise Operator : simulink/Logic and Bit Operations/Bitwise Operator  logicop=AND  UseBitMask=on  BitMask=1  BitMaskRealWorld=Stored Integer
  Compare To Zero : simulink/Logic and Bit Operations/Compare To Zero  SystemSampleTime=-1  relop===  LogicOutDataTypeMode=uint8  ZeroCross=off
  Counter Free-Running : simulink/Sources/Counter Free-Running  SystemSampleTime=-1  NumBits=32  tsamp=-1
  Out1 : Outport  InitialOutput=0
  wires:
  Counter Free-Running/1 -> Bitwise Operator/1
  Bitwise Operator/1 -> Compare To Zero/1
  Compare To Zero/1 -> Out1/1

== system amg_high_precision_rtc/STM32F4/DS3231 Configure/Enabled Subsystem/Debouce3/Enabled Subsystem4 ==
  Enable : EnablePort  PropagateVarSize=During execution
  Counter Free-Running : simulink/Sources/Counter Free-Running  SystemSampleTime=-1  NumBits=32  tsamp=-1
  Out1 : Outport  InitialOutput=0
  wires:
  Counter Free-Running/1 -> Out1/1

== system amg_high_precision_rtc/STM32F4/DS3231 Configure/Enabled Subsystem/Debouce3/Enabled Subsystem5 ==
  Enable : EnablePort  PropagateVarSize=During execution
  Counter Free-Running : simulink/Sources/Counter Free-Running  SystemSampleTime=-1  NumBits=32  tsamp=-1
  Out1 : Outport  InitialOutput=0
  wires:
  Counter Free-Running/1 -> Out1/1

== system amg_high_precision_rtc/STM32F4/DS3231 Configure/Enabled Subsystem/Generate Mode ID/Enabled Subsystem2 ==
  Enable : EnablePort  PropagateVarSize=During execution
  Bitwise Operator : simulink/Logic and Bit Operations/Bitwise Operator  logicop=AND  UseBitMask=on  BitMask=7  BitMaskRealWorld=Stored Integer
  Counter Free-Running : simulink/Sources/Counter Free-Running  SystemSampleTime=-1  NumBits=16  tsamp=-1
  Out1 : Outport  InitialOutput=0
  wires:
  Counter Free-Running/1 -> Bitwise Operator/1
  Bitwise Operator/1 -> Out1/1

== system amg_high_precision_rtc/STM32F4/DS3231 Configure/Enabled Subsystem/Subsystem/DS3231 Get Date ==
  Slave Address : Inport
  Compare To Zero : simulink/Logic and Bit Operations/Compare To Zero  SystemSampleTime=-1  relop===  LogicOutDataTypeMode=uint8  ZeroCross=off
  Convert : Subsystem  TreatAsAtomicUnit=on
  I2C Master Read/Write : S-Function  FunctionName=stm32f4_i2c  Parameters=configuration,module,transfer,clkspeed,timeout,sdapin,sclpin,writecount,readcount,inputtypearray,outputtypearray,confstr,sampletime,sampletimestr,blockid  SFunctionDeploymentMode=off  EnableBusSupport=off  mask(stm32f4_i2c){configuration=Transaction, module=1, lastmodule=3, transfer=Blocking, dutycycle=TLow/THigh = 2, clkspeed=400, timeout=25, writecount=1, readcount=4, sdapin=C9, sclpin=A8, waitwritetime=0, inputtypearray=[2 3 3], outputtypearray=[5 3 3 3 3 3], confstr=["C","9","A","8","1","1","6","0","I2C_DutyCycle_2","0"], sampletime=-1, sampletimestr=0.01, blockid=configureDS3231ConfigureEnabledSubsystemSubsystemDS3231GetDateI2CMasterReadWrite}
      mask prompts: module "I2C Module"; lastmodule "Last module"; transfer "Transfer mode"; dutycycle "Duty cycle in fast mode"; clkspeed "Clock speed (kHz)"; timeout "Timeout (ms)"; writecount "Bytes write count"; readcount "Bytes read count"; sdapin "SDA pin"; sclpin "SCL pin"; waitwritetime "Wait write time (ms), default is 0"; inputtypearray "Input type array"; outputtypearray "Output type array"; confstr "Configuration string"; sampletime "Sample time (sec)"; sampletimestr "Compiled sample time (sec) in string"
      mask init:
      | stm32f4_i2c_callback('init');
      mask Help: web(fullfile(waijungdocroot,'stm32f4_i2c_readwrite.htm'), '-browser')
      mask TypeOptions configuration: Setup | Transaction
      mask Callback configuration: stm32f4_i2c_callback('configuration');
      mask TypeOptions module: 1 | 2 | 3
      mask Callback module: stm32f4_i2c_callback('module');
      mask TypeOptions transfer: Blocking | Non-blocking
      mask TypeOptions dutycycle: TLow/THigh = 16/9 | TLow/THigh = 2
      mask Callback dutycycle: stm32f4_i2c_callback('dutycycle');
      mask Callback writecount: stm32f4_i2c_callback('writecount');
      mask Callback readcount: stm32f4_i2c_callback('readcount');
      mask TypeOptions sdapin: - | C9
      mask Callback sdapin: stm32f4_i2c_callback('sdapin');
      mask TypeOptions sclpin: - | A8
      mask Callback sclpin: stm32f4_i2c_callback('sclpin');
      mask Callback confstr: stm32f4_i2c_callback('confstr');
      mask Callback sampletime: stm32f4_i2c_callback('sampletime');
      mask Callback sampletimestr: stm32f4_i2c_callback('sampletimestr');
      mask Callback blockid: stm32f4_i2c_callback('blockid');
      mask Display: text(0.5, 0.5, 'Module: I2C1\nTransfer: Blocking\nWrite: 1 bytes\nRead: 4 bytes\nTs (sec): 0.01','ver','middle','hor','center');port_label('input', 1,'SlvAddr');port_label('input', 2,'Wr0 (uint8)');port_label('output', 1,'Status');port_label('output', 2,'Rd0 (uint8)');port_label('output', 3,'Rd1 (uint8)');port_label('output', 4,'Rd2 (uint8)');port_label('output', 5,'Rd3 (uint8)');
  REG_DATE : Constant  Value=hex2dec('03')  OutDataTypeStr=uint8
  Status : Outport
  Day : Outport  Port=2
  Date : Outport  Port=3
  Month : Outport  Port=4
  Year : Outport  Port=5
  wires:
  Convert/3(Month) -> Month/1
  Convert/4(Year) -> Year/1
  Convert/2(Date) -> Date/1
  Convert/1(Day) -> Day/1
  I2C Master Read/Write/5 -> Convert/4(In4)
  REG_DATE/1 -> I2C Master Read/Write/2
  Slave Address/1 -> I2C Master Read/Write/1
  I2C Master Read/Write/1 -> Compare To Zero/1
  Compare To Zero/1 -> Convert/Enable, Status/1
  I2C Master Read/Write/2 -> Convert/1(In1)
  I2C Master Read/Write/3 -> Convert/2(In2)
  I2C Master Read/Write/4 -> Convert/3(In3)

== system amg_high_precision_rtc/STM32F4/DS3231 Configure/Enabled Subsystem/Subsystem/DS3231 Get Time ==
  Slave Address : Inport
  Compare To Zero : simulink/Logic and Bit Operations/Compare To Zero  SystemSampleTime=-1  relop===  LogicOutDataTypeMode=uint8  ZeroCross=off
  Convert : Subsystem  TreatAsAtomicUnit=on
  Data Type Conversion{,1..3} (4 alike) : DataTypeConversion  OutDataTypeStr=uint8
  I2C Master Read/Write : S-Function  FunctionName=stm32f4_i2c  Parameters=configuration,module,transfer,clkspeed,timeout,sdapin,sclpin,writecount,readcount,inputtypearray,outputtypearray,confstr,sampletime,sampletimestr,blockid  SFunctionDeploymentMode=off  EnableBusSupport=off  mask(stm32f4_i2c){configuration=Transaction, module=1, lastmodule=3, transfer=Blocking, dutycycle=TLow/THigh = 2, clkspeed=400, timeout=25, writecount=1, readcount=3, sdapin=C9, sclpin=A8, waitwritetime=0, inputtypearray=[2 3 3], outputtypearray=[4 3 3 3 3], confstr=["C","9","A","8","1","1","6","0","I2C_DutyCycle_2","0"], sampletime=-1, sampletimestr=0.01, blockid=configureDS3231ConfigureEnabledSubsystemSubsystemDS3231GetTimeI2CMasterReadWrite}
      mask prompts: module "I2C Module"; lastmodule "Last module"; transfer "Transfer mode"; dutycycle "Duty cycle in fast mode"; clkspeed "Clock speed (kHz)"; timeout "Timeout (ms)"; writecount "Bytes write count"; readcount "Bytes read count"; sdapin "SDA pin"; sclpin "SCL pin"; waitwritetime "Wait write time (ms), default is 0"; inputtypearray "Input type array"; outputtypearray "Output type array"; confstr "Configuration string"; sampletime "Sample time (sec)"; sampletimestr "Compiled sample time (sec) in string"
      mask init:
      | stm32f4_i2c_callback('init');
      mask Help: web(fullfile(waijungdocroot,'stm32f4_i2c_readwrite.htm'), '-browser')
      mask TypeOptions configuration: Setup | Transaction
      mask Callback configuration: stm32f4_i2c_callback('configuration');
      mask TypeOptions module: 1 | 2 | 3
      mask Callback module: stm32f4_i2c_callback('module');
      mask TypeOptions transfer: Blocking | Non-blocking
      mask TypeOptions dutycycle: TLow/THigh = 16/9 | TLow/THigh = 2
      mask Callback dutycycle: stm32f4_i2c_callback('dutycycle');
      mask Callback writecount: stm32f4_i2c_callback('writecount');
      mask Callback readcount: stm32f4_i2c_callback('readcount');
      mask TypeOptions sdapin: - | C9
      mask Callback sdapin: stm32f4_i2c_callback('sdapin');
      mask TypeOptions sclpin: - | A8
      mask Callback sclpin: stm32f4_i2c_callback('sclpin');
      mask Callback confstr: stm32f4_i2c_callback('confstr');
      mask Callback sampletime: stm32f4_i2c_callback('sampletime');
      mask Callback sampletimestr: stm32f4_i2c_callback('sampletimestr');
      mask Callback blockid: stm32f4_i2c_callback('blockid');
      mask Display: text(0.5, 0.5, 'Module: I2C1\nTransfer: Blocking\nWrite: 1 bytes\nRead: 3 bytes\nTs (sec): 0.01','ver','middle','hor','center');port_label('input', 1,'SlvAddr');port_label('input', 2,'Wr0 (uint8)');port_label('output', 1,'Status');port_label('output', 2,'Rd0 (uint8)');port_label('output', 3,'Rd1 (uint8)');port_label('output', 4,'Rd2 (uint8)');
  REG_TIME : Constant  Value=hex2dec('00')  OutDataTypeStr=uint8
  Status : Outport
  Hour : Outport  Port=2
  Minute : Outport  Port=3
  Second : Outport  Port=4
  AM/PM : Outport  Port=5
  wires:
  Data Type Conversion3/1 -> AM/PM/1
  Data Type Conversion2/1 -> Second/1
  Data Type Conversion1/1 -> Minute/1
  Data Type Conversion/1 -> Hour/1
  Convert/4(AM/PM) -> Data Type Conversion3/1
  Convert/1(Hour) -> Data Type Conversion/1
  Convert/2(Minute) -> Data Type Conversion1/1
  Convert/3(Second) -> Data Type Conversion2/1
  I2C Master Read/Write/4 -> Convert/3(In3)
  I2C Master Read/Write/3 -> Convert/2(In2)
  I2C Master Read/Write/2 -> Convert/1(In1)
  Compare To Zero/1 -> Status/1, Convert/Enable
  I2C Master Read/Write/1 -> Compare To Zero/1
  Slave Address/1 -> I2C Master Read/Write/1
  REG_TIME/1 -> I2C Master Read/Write/2

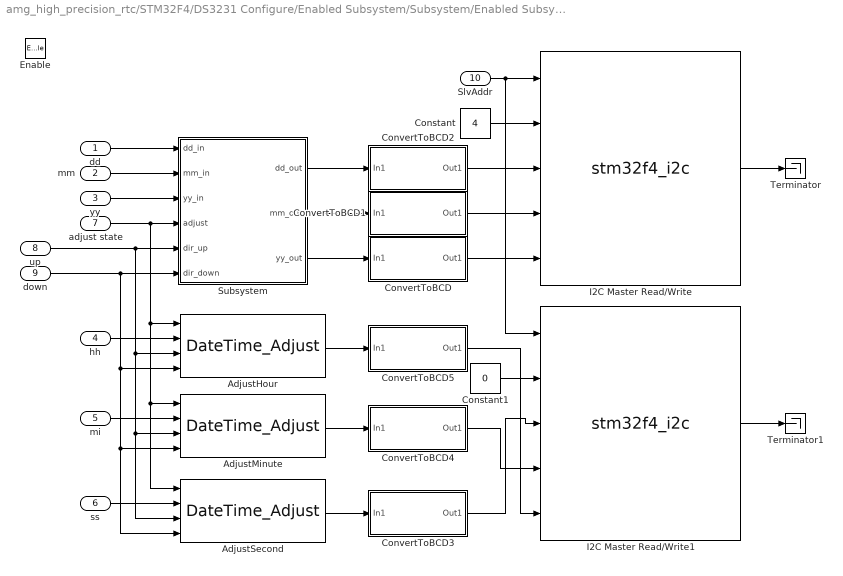
== system amg_high_precision_rtc/STM32F4/DS3231 Configure/Enabled Subsystem/Subsystem/Enabled Subsystem ==
  dd : Inport
  mm : Inport  Port=2
  yy : Inport  Port=3
  hh : Inport  Port=4
  mi : Inport  Port=5
  ss : Inport  Port=6
  adjust state : Inport  Port=7
  up : Inport  Port=8
  down : Inport  Port=9
  SlvAddr : Inport  Port=10
  Enable : EnablePort  PropagateVarSize=During execution
  AdjustHour : amg_high_precision_rtc/DateTime_Adjust  SystemSampleTime=-1  state=3  max=23  min=0
  AdjustMinute : amg_high_precision_rtc/DateTime_Adjust  SystemSampleTime=-1  state=4  max=59  min=0
  AdjustSecond : amg_high_precision_rtc/DateTime_Adjust  SystemSampleTime=-1  state=5  max=59  min=0
  Constant : Constant  Value=4  OutDataTypeStr=uint8
  Constant1 : Constant  Value=0  OutDataTypeStr=uint8
  ConvertToBCD : Subsystem  TreatAsAtomicUnit=on
      settings: RTWFcnNameOpts=Use subsystem name  RTWFileNameOpts=Use function name
      mask Display: disp('Dec-to-BCD');
  ConvertToBCD1 : Subsystem  TreatAsAtomicUnit=on
      settings: RTWFcnNameOpts=Use subsystem name  RTWFileNameOpts=Use function name
      mask Display: disp('Dec-to-BCD');
  ConvertToBCD2 : Subsystem  TreatAsAtomicUnit=on
      settings: RTWFcnNameOpts=Use subsystem name  RTWFileNameOpts=Use function name
      mask Display: disp('Dec-to-BCD');
  ConvertToBCD3 : Subsystem  TreatAsAtomicUnit=on
      settings: RTWFcnNameOpts=Use subsystem name  RTWFileNameOpts=Use function name
      mask Display: disp('Dec-to-BCD');
  ConvertToBCD4 : Subsystem  TreatAsAtomicUnit=on
      settings: RTWFcnNameOpts=Use subsystem name  RTWFileNameOpts=Use function name
      mask Display: disp('Dec-to-BCD');
  ConvertToBCD5 : Subsystem  TreatAsAtomicUnit=on
      settings: RTWFcnNameOpts=Use subsystem name  RTWFileNameOpts=Use function name
      mask Display: disp('Dec-to-BCD');
  I2C Master Read/Write : S-Function  FunctionName=stm32f4_i2c  Parameters=configuration,module,transfer,clkspeed,timeout,sdapin,sclpin,writecount,readcount,inputtypearray,outputtypearray,confstr,sampletime,sampletimestr,blockid  SFunctionDeploymentMode=off  EnableBusSupport=off  mask(stm32f4_i2c){configuration=Transaction, module=1, lastmodule=3, transfer=Blocking, dutycycle=TLow/THigh = 2, clkspeed=400, timeout=25, writecount=4, readcount=0, sdapin=C9, sclpin=A8, waitwritetime=0, inputtypearray=[5 3 3 3 3 3], outputtypearray=[1 3], confstr=["C","9","A","8","1","1","6","0","I2C_DutyCycle_2","0"], sampletime=-1, sampletimestr=0.01, blockid=configureDS3231ConfigureEnabledSubsystemSubsystemEnabledSubsystemI2CMasterReadWrite}
      mask prompts: module "I2C Module"; lastmodule "Last module"; transfer "Transfer mode"; dutycycle "Duty cycle in fast mode"; clkspeed "Clock speed (kHz)"; timeout "Timeout (ms)"; writecount "Bytes write count"; readcount "Bytes read count"; sdapin "SDA pin"; sclpin "SCL pin"; waitwritetime "Wait write time (ms), default is 0"; inputtypearray "Input type array"; outputtypearray "Output type array"; confstr "Configuration string"; sampletime "Sample time (sec)"; sampletimestr "Compiled sample time (sec) in string"
      mask init:
      | stm32f4_i2c_callback('init');
      mask Help: web(fullfile(waijungdocroot,'stm32f4_i2c_readwrite.htm'), '-browser')
      mask TypeOptions configuration: Setup | Transaction
      mask Callback configuration: stm32f4_i2c_callback('configuration');
      mask TypeOptions module: 1 | 2 | 3
      mask Callback module: stm32f4_i2c_callback('module');
      mask TypeOptions transfer: Blocking | Non-blocking
      mask TypeOptions dutycycle: TLow/THigh = 16/9 | TLow/THigh = 2
      mask Callback dutycycle: stm32f4_i2c_callback('dutycycle');
      mask Callback writecount: stm32f4_i2c_callback('writecount');
      mask Callback readcount: stm32f4_i2c_callback('readcount');
      mask TypeOptions sdapin: - | C9
      mask Callback sdapin: stm32f4_i2c_callback('sdapin');
      mask TypeOptions sclpin: - | A8
      mask Callback sclpin: stm32f4_i2c_callback('sclpin');
      mask Callback confstr: stm32f4_i2c_callback('confstr');
      mask Callback sampletime: stm32f4_i2c_callback('sampletime');
      mask Callback sampletimestr: stm32f4_i2c_callback('sampletimestr');
      mask Callback blockid: stm32f4_i2c_callback('blockid');
      mask Display: text(0.5, 0.5, 'Module: I2C1\nTransfer: Blocking\nWrite: 4 bytes\nRead: 0 bytes\nTs (sec): 0.01','ver','middle','hor','center');port_label('input', 1,'SlvAddr');port_label('input', 2,'Wr0 (uint8)');port_label('input', 3,'Wr1 (uint8)');port_label('input', 4,'Wr2 (uint8)');port_label('input', 5,'Wr3 (uint8)');port_label('output', 1,'Status');
  I2C Master Read/Write1 : S-Function  FunctionName=stm32f4_i2c  Parameters=configuration,module,transfer,clkspeed,timeout,sdapin,sclpin,writecount,readcount,inputtypearray,outputtypearray,confstr,sampletime,sampletimestr,blockid  SFunctionDeploymentMode=off  EnableBusSupport=off  mask(stm32f4_i2c){configuration=Transaction, module=1, lastmodule=3, transfer=Blocking, dutycycle=TLow/THigh = 2, clkspeed=400, timeout=25, writecount=4, readcount=0, sdapin=C9, sclpin=A8, waitwritetime=0, inputtypearray=[5 3 3 3 3 3], outputtypearray=[1 3], confstr=["C","9","A","8","1","1","6","0","I2C_DutyCycle_2","0"], sampletime=-1, sampletimestr=0.01, blockid=configureDS3231ConfigureEnabledSubsystemSubsystemEnabledSubsystemI2CMasterReadWrite1}
      mask prompts: module "I2C Module"; lastmodule "Last module"; transfer "Transfer mode"; dutycycle "Duty cycle in fast mode"; clkspeed "Clock speed (kHz)"; timeout "Timeout (ms)"; writecount "Bytes write count"; readcount "Bytes read count"; sdapin "SDA pin"; sclpin "SCL pin"; waitwritetime "Wait write time (ms), default is 0"; inputtypearray "Input type array"; outputtypearray "Output type array"; confstr "Configuration string"; sampletime "Sample time (sec)"; sampletimestr "Compiled sample time (sec) in string"
      mask init:
      | stm32f4_i2c_callback('init');
      mask Help: web(fullfile(waijungdocroot,'stm32f4_i2c_readwrite.htm'), '-browser')
      mask TypeOptions configuration: Setup | Transaction
      mask Callback configuration: stm32f4_i2c_callback('configuration');
      mask TypeOptions module: 1 | 2 | 3
      mask Callback module: stm32f4_i2c_callback('module');
      mask TypeOptions transfer: Blocking | Non-blocking
      mask TypeOptions dutycycle: TLow/THigh = 16/9 | TLow/THigh = 2
      mask Callback dutycycle: stm32f4_i2c_callback('dutycycle');
      mask Callback writecount: stm32f4_i2c_callback('writecount');
      mask Callback readcount: stm32f4_i2c_callback('readcount');
      mask TypeOptions sdapin: - | C9
      mask Callback sdapin: stm32f4_i2c_callback('sdapin');
      mask TypeOptions sclpin: - | A8
      mask Callback sclpin: stm32f4_i2c_callback('sclpin');
      mask Callback confstr: stm32f4_i2c_callback('confstr');
      mask Callback sampletime: stm32f4_i2c_callback('sampletime');
      mask Callback sampletimestr: stm32f4_i2c_callback('sampletimestr');
      mask Callback blockid: stm32f4_i2c_callback('blockid');
      mask Display: text(0.5, 0.5, 'Module: I2C1\nTransfer: Blocking\nWrite: 4 bytes\nRead: 0 bytes\nTs (sec): 0.01','ver','middle','hor','center');port_label('input', 1,'SlvAddr');port_label('input', 2,'Wr0 (uint8)');port_label('input', 3,'Wr1 (uint8)');port_label('input', 4,'Wr2 (uint8)');port_label('input', 5,'Wr3 (uint8)');port_label('output', 1,'Status');
  Subsystem : Subsystem
  Terminator : Terminator
  Terminator1 : Terminator
  wires:
  dd/1 -> Subsystem/1(dd_in)
  mm/1 -> Subsystem/2(mm_in)
  yy/1 -> Subsystem/3(yy_in)
  adjust state/1 -> Subsystem/4(adjust), AdjustHour/1, AdjustMinute/1, AdjustSecond/1
  up/1 -> Subsystem/5(dir_up), AdjustHour/3, AdjustMinute/3, AdjustSecond/3
  down/1 -> Subsystem/6(dir_down), AdjustHour/4, AdjustMinute/4, AdjustSecond/4
  SlvAddr/1 -> I2C Master Read/Write/1, I2C Master Read/Write1/1
  Subsystem/1(dd_out) -> ConvertToBCD2/1(In1)
  Subsystem/2(mm_out) -> ConvertToBCD1/1(In1)
  Subsystem/3(yy_out) -> ConvertToBCD/1(In1)
  Constant/1 -> I2C Master Read/Write/2
  I2C Master Read/Write/1 -> Terminator/1
  ConvertToBCD2/1(Out1) -> I2C Master Read/Write/3
  ConvertToBCD1/1(Out1) -> I2C Master Read/Write/4
  ConvertToBCD/1(Out1) -> I2C Master Read/Write/5
  ss/1 -> AdjustSecond/2
  mi/1 -> AdjustMinute/2
  hh/1 -> AdjustHour/2
  Constant1/1 -> I2C Master Read/Write1/2
  I2C Master Read/Write1/1 -> Terminator1/1
  ConvertToBCD4/1(Out1) -> I2C Master Read/Write1/4
  AdjustHour/1 -> ConvertToBCD5/1(In1)
  AdjustMinute/1 -> ConvertToBCD4/1(In1)
  AdjustSecond/1 -> ConvertToBCD3/1(In1)
  ConvertToBCD5/1(Out1) -> I2C Master Read/Write1/5
  ConvertToBCD3/1(Out1) -> I2C Master Read/Write1/3

== system amg_high_precision_rtc/Soft I2C/Soft-DS3231 Configure/Enabled Subsystem/Debouce1/Enabled Subsystem ==
  Enable : EnablePort  PropagateVarSize=During execution
  Counter Free-Running : simulink/Sources/Counter Free-Running  SystemSampleTime=-1  NumBits=32  tsamp=-1
  Out1 : Outport  InitialOutput=0
  wires:
  Counter Free-Running/1 -> Out1/1

== system amg_high_precision_rtc/Soft I2C/Soft-DS3231 Configure/Enabled Subsystem/Debouce1/Enabled Subsystem1 ==
  Enable : EnablePort  PropagateVarSize=During execution
  Bitwise Operator : simulink/Logic and Bit Operations/Bitwise Operator  logicop=AND  UseBitMask=on  BitMask=1  BitMaskRealWorld=Stored Integer
  Compare To Zero : simulink/Logic and Bit Operations/Compare To Zero  SystemSampleTime=-1  relop===  LogicOutDataTypeMode=uint8  ZeroCross=off
  Counter Free-Running : simulink/Sources/Counter Free-Running  SystemSampleTime=-1  NumBits=32  tsamp=-1
  Out1 : Outport  InitialOutput=0
  wires:
  Compare To Zero/1 -> Out1/1
  Bitwise Operator/1 -> Compare To Zero/1
  Counter Free-Running/1 -> Bitwise Operator/1

== system amg_high_precision_rtc/Soft I2C/Soft-DS3231 Configure/Enabled Subsystem/Debouce1/Enabled Subsystem4 ==
  Enable : EnablePort  PropagateVarSize=During execution
  Counter Free-Running : simulink/Sources/Counter Free-Running  SystemSampleTime=-1  NumBits=32  tsamp=-1
  Out1 : Outport  InitialOutput=0
  wires:
  Counter Free-Running/1 -> Out1/1

== system amg_high_precision_rtc/Soft I2C/Soft-DS3231 Configure/Enabled Subsystem/Debouce1/Enabled Subsystem5 ==
  Enable : EnablePort  PropagateVarSize=During execution
  Counter Free-Running : simulink/Sources/Counter Free-Running  SystemSampleTime=-1  NumBits=32  tsamp=-1
  Out1 : Outport  InitialOutput=0
  wires:
  Counter Free-Running/1 -> Out1/1

== system amg_high_precision_rtc/Soft I2C/Soft-DS3231 Configure/Enabled Subsystem/Debouce2/Enabled Subsystem ==
  Enable : EnablePort  PropagateVarSize=During execution
  Counter Free-Running : simulink/Sources/Counter Free-Running  SystemSampleTime=-1  NumBits=32  tsamp=-1
  Out1 : Outport  InitialOutput=0
  wires:
  Counter Free-Running/1 -> Out1/1
